simulink model "FullyConnectedMMG"  (R2020b)
settings: Solver=ode3  StartTime=0.0  StopTime=TimeS  FixedStep=Ts  RelTol=1e-3
values from neighbouring files (symbols this model uses):
  fr = 60    [MMG_Parameters.m]
  Lgs = 600e-6    (= 0.0006)    [MMG_Parameters.m]
  MaxWind = 18    [MMG_Parameters.m]
  MicroVol = 575    [MMG_Parameters.m]
  MinWind = 3    [MMG_Parameters.m]
  NomVol = 600    [MMG_Parameters.m]
  NomWind = 10    [MMG_Parameters.m]
  Pnombb = 400    [MMG_Parameters.m]
  PnomDG = 150e3    (= 150000)    [MMG_Parameters.m]
  PnomWT = 400e3    (= 400000)    [MMG_Parameters.m]
  Rgs = 20e-6    (= 2e-05)    [MMG_Parameters.m]
  RtCapM1 = (5.1)*1e-1    (= 0.51)    [MMG_Parameters.m]
  RtCapM2 = (5.1)*1e-1    (= 0.51)    [MMG_Parameters.m]
  SOC = [70,80,75,65]    [MMG_Parameters.m]
  Ts = 8e-4    (= 0.0008)    [MMG_Parameters.m]    (also in SolveMONO.m = 0.005)
  Vgrid = 25e3    (= 25000)    [MMG_Parameters.m]
  VMic = 575    [MMG_Parameters.m]
  Vs = 120e3    (= 120000)    [MMG_Parameters.m]
undefined symbols (not defined in the file or in its folder): DiscIntNeverNeededParam
libraries: powerlib x64, simulink x24, powerlib_meascontrol x16
(part 1 of 5)
settings Model: SimulationMode=accelerator  Creator=jlesage  LastModifiedBy=ferna
settings DataIOCC: ReturnWorkspaceOutputs=off
settings OptimizationCC: EfficientMapNaN2IntZero=off
settings DebuggingCC: UnconnectedInputMsg=none  UnconnectedOutputMsg=none  UnconnectedLineMsg=none  ArithmeticOperatorsInVariantConditions=warning
settings HardwareCC: TargetBitPerPointer=64  TargetBitPerSizeT=64  TargetBitPerPtrDiffT=64  TargetLongLongMode=on  TargetIntDivRoundTo=Zero  TargetEndianess=LittleEndian  TargetWordSize=64  TargetHWDeviceType=MATLAB Host  ProdEqTarget=off
settings SFSimCC: SimUseLocalCustomCode=off  CustomCodeUndefinedFunction=UseInterfaceOnly
settings CodeAppCC: MaxIdLength=128
settings GRTTargetCC: CombineOutputUpdateFcns=off  GRTInterface=on

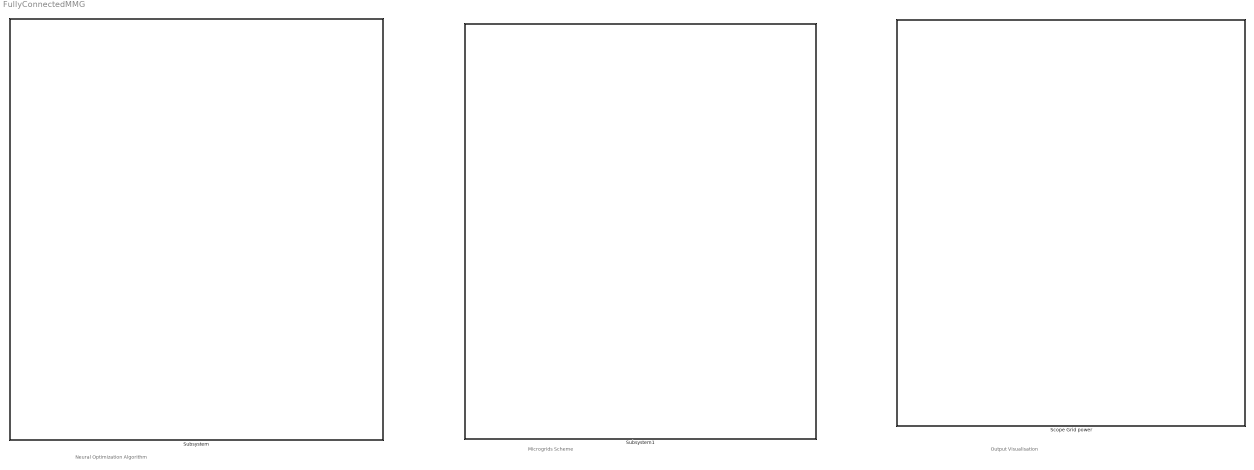
== system FullyConnectedMMG ==
  note: Output Visualisation
  note: Microgrids Scheme
  note: Neural Optimization Algorithm
  Scope Grid power : Subsystem
  Subsystem : Subsystem
  Subsystem1 : Subsystem

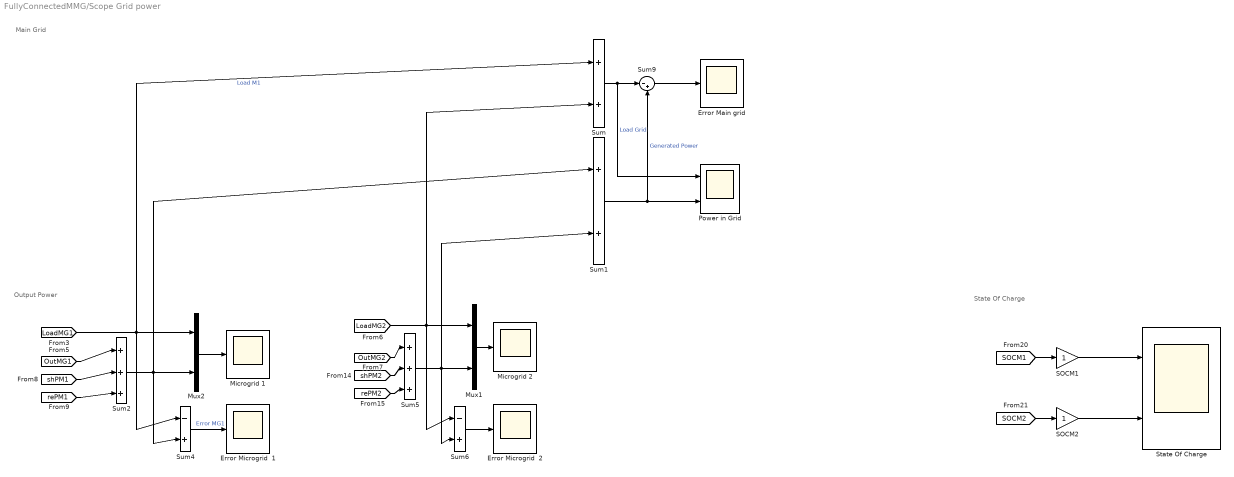
== system FullyConnectedMMG/Scope Grid power ==
  note: State Of Charge
  note: Output Power
  note: Main Grid
  Error Main grid : Scope
  Error Microgrid  1 : Scope
  Error Microgrid  2 : Scope
  Microgrid 1 : Scope
  Microgrid 2 : Scope
  Mux1 : Mux  Inputs=2
  Mux2 : Mux  Inputs=2
  Power in Grid : Scope  NumInputPorts=2
  SOCM1 : Gain
  SOCM2 : Gain
  State Of Charge : Scope  NumInputPorts=2
  Sum : Sum  Inputs=|++
  Sum1 : Sum  Inputs=|++
  Sum2 : Sum  Inputs=|+++
  Sum4 : Sum  Inputs=|-+
  Sum5 : Sum  Inputs=|+++
  Sum6 : Sum  Inputs=|-+
  Sum9 : Sum  Inputs=|-+
  wires:
  Sum5/1 -> Sum6/2, Mux1/2, Sum1/2
  Sum1/1 -> Power in Grid/2, Sum9/2  "Generated Power"
  Sum/1 -> Power in Grid/1, Sum9/1  "Load Grid"
  Mux2/1 -> Microgrid 1/1
  [LoadMG1] -> Sum/1, Mux2/1, Sum4/1  "Load M1"
  [LoadMG2] -> Sum6/1, Mux1/1, Sum/2
  Mux1/1 -> Microgrid 2/1
  Sum2/1 -> Sum4/2, Sum1/1, Mux2/2
  Sum4/1 -> Error Microgrid  1/1  "Error MG1"
  Sum6/1 -> Error Microgrid  2/1
  [SOCM1] -> SOCM1/1
  [SOCM2] -> SOCM2/1
  Sum9/1 -> Error Main grid/1
  SOCM1/1 -> State Of Charge/1
  SOCM2/1 -> State Of Charge/2
  [OutMG1] -> Sum2/1
  [OutMG2] -> Sum5/1
  [shPM1] -> Sum2/2
  [rePM1] -> Sum2/3
  [shPM2] -> Sum5/2
  [rePM2] -> Sum5/3

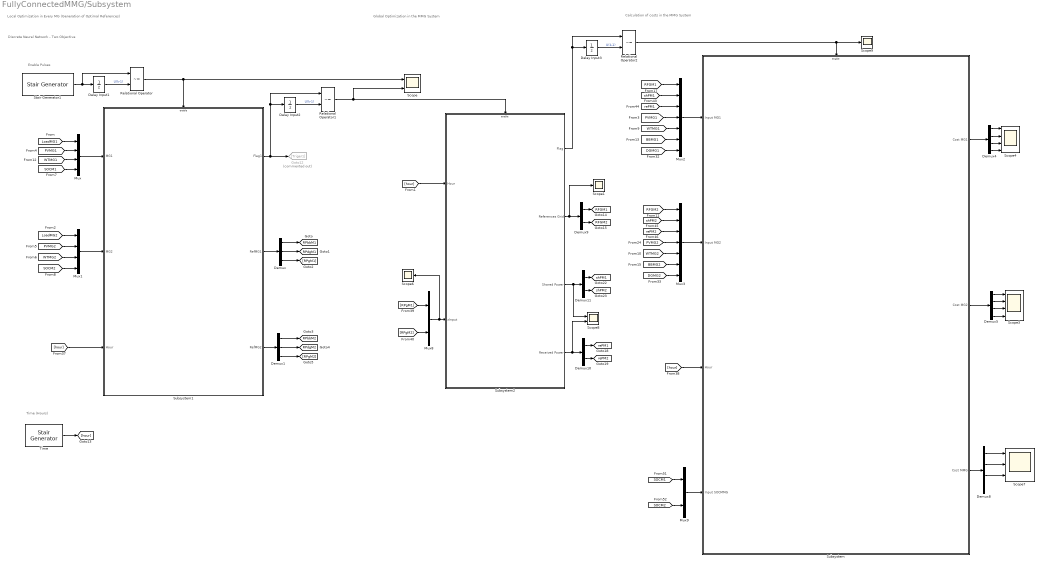
== system FullyConnectedMMG/Subsystem ==
  note: Enable Pulses
  note: Local Optimization in Every MG (Generation of Optimal References)
  note: Discrete Neural Network - Two Objective
  note: Calculation of costs in the MMG System
  note: Global Optimization in the MMG System
  note: Time (Hours)
  Delay Input1 : UnitDelay  Description=Store in Global RAM  DisableCoverage=on  SampleTime=-1  HasFrameUpgradeWarning=on
  Delay Input2 : UnitDelay  Description=Store in Global RAM  DisableCoverage=on  SampleTime=-1  HasFrameUpgradeWarning=on
  Delay Input3 : UnitDelay  Description=Store in Global RAM  DisableCoverage=on  SampleTime=-1  HasFrameUpgradeWarning=on
  Demux : Demux  Outputs=3
  Demux1 : Demux  Outputs=3
  Demux10 : Demux  Outputs=2
  Demux11 : Demux  Outputs=2
  Demux4 : Demux
  Demux5 : Demux
  Demux8 : Demux
  Demux9 : Demux  Outputs=2
  Goto12 : Goto  Commented=on  GotoTag=Triger1
  Mux : Mux
  Mux1 : Mux
  Mux2 : Mux  Inputs=7
  Mux3 : Mux  Inputs=7
  Mux8 : Mux  Inputs=2
  Mux9 : Mux  Inputs=2
  Relational Operator : RelationalOperator  Operator=~=  OutDataTypeStr=fixdt(0, 8)  ZeroCross=off  RndMeth=Nearest
  Relational Operator1 : RelationalOperator  Operator=~=  OutDataTypeStr=fixdt(0, 8)  ZeroCross=off  RndMeth=Nearest
  Relational Operator2 : RelationalOperator  Operator=~=  OutDataTypeStr=fixdt(0, 8)  ZeroCross=off  RndMeth=Nearest
  Scope : Scope  NumInputPorts=2
  Scope1 : Scope
  Scope3 : Scope  NumInputPorts=4
  Scope4 : Scope  NumInputPorts=4
  Scope6 : Scope
  Scope7 : Scope  NumInputPorts=3
  Scope8 : Scope  NumInputPorts=2
  Scope9 : Scope
  Stair Generator1 : powerlib_meascontrol/Pulse & Signal Generators/Stair Generator  t=[0, 1, 2, 3, 4, 5, 6, 7, 8, 9, 10, 11, 12, 13, 14, 15, 16, 17, 18, 19, 20, 21, 22, 23]+0.04  e=[1,2,3,4,5,6,7,8,9,10,11,12,13,14,15,16,17,18,19,20,21,22,23,24]  Ts=Ts
  Subsystem : Subsystem
  Subsystem1 : Subsystem
  Subsystem2 : Subsystem
  Time : powerlib_meascontrol/Pulse & Signal Generators/Stair Generator  t=[0.5,1.5,2.5,3.5,4.5,5.5,6.5,7.5,8.5,9.5,10.5,11.5,12.5,13.5,14.5,15.5,16.5,17.5,18.5,19.5,20.5,21.5,22.5,23.5]  e=[1,2,3,4,5,6,7,8,9,10,11,12,13,14,15,16,17,18,19,20,21,22,23,24]  Ts=0
  tag scope: RFGM1=global, RFGM2=global, RPbbM1=global, RPbbM2=global, RPdgM1=global, RPdgM2=global, rePM1=global, rePM2=global, shPM1=global, shPM2=global
  wires:
  Demux1/2 -> [RPdgM2]
  [SOCM2] -> Mux1/4
  Demux/1 -> [RPbbM1]
  [LoadMG1] -> Mux/1
  [PVMG1] -> Mux/2
  Demux/2 -> [RPdgM1]
  Demux1/3 -> [RPgM2]
  Demux1/1 -> [RPbbM2]
  [WTMG2] -> Mux1/3
  [PVMG2] -> Mux1/2
  [WTMG1] -> Mux/3
  [SOCM1] -> Mux/4
  Demux/3 -> [RPgM1]
  [LoadMG2] -> Mux1/1
  Mux2/1 -> Subsystem/1(Input MG1)
  [hour] -> Subsystem/3(Hour)
  Demux4/1 -> Scope4/1
  Demux4/2 -> Scope4/2
  Subsystem/1(Cost MG1) -> Demux4/1
  Demux5/2 -> Scope3/2
  Demux5/1 -> Scope3/1
  Subsystem/2(Cost MG2) -> Demux5/1
  Demux8/3 -> Scope7/3
  Demux8/1 -> Scope7/1
  Demux8/2 -> Scope7/2
  Subsystem/3(Cost MMG) -> Demux8/1
  Stair Generator1/1 -> Relational Operator/1, Delay Input1/1
  Delay Input1/1 -> Relational Operator/2  "U(k-1)"
  Relational Operator/1 -> Subsystem1/Enable, Scope/1
  Mux/1 -> Subsystem1/1(MG1)
  Mux1/1 -> Subsystem1/2(MG2)
  [hour] -> Subsystem1/3(Hour)
  Subsystem1/1(Flag1) -> Relational Operator1/1, Delay Input2/1, Goto12/1
  Subsystem1/2(RefMG1) -> Demux/1
  Subsystem1/3(RefMG2) -> Demux1/1
  Time/1 -> [hour]
  Relational Operator2/1 -> Scope9/1, Subsystem/Enable
  [RPgM1] -> Mux8/1
  [RPgM2] -> Mux8/2
  [hour] -> Subsystem2/1(Hour)
  Mux8/1 -> Scope6/1, Subsystem2/2(xInput)
  Delay Input2/1 -> Relational Operator1/2  "U(k-1)"
  Relational Operator1/1 -> Subsystem2/Enable, Scope/2
  Subsystem2/2(References Grid) -> Demux9/1, Scope1/1
  Demux9/1 -> [RFGM1]
  Demux9/2 -> [RFGM2]
  Demux10/2 -> [rePM2]
  Demux10/1 -> [rePM1]
  Subsystem2/3(Shared Power) -> Scope8/1, Demux11/1
  Subsystem2/4(Received Power) -> Scope8/2, Demux10/1
  Demux11/1 -> [shPM1]
  Demux11/2 -> [shPM2]
  [RFGM1] -> Mux2/1
  [rePM1] -> Mux2/3
  [shPM1] -> Mux2/2
  [PVMG1] -> Mux2/4
  [WTMG1] -> Mux2/5
  [BBMG1] -> Mux2/6
  [DGMG1] -> Mux2/7
  Mux3/1 -> Subsystem/2(Input MG2)
  [DGMG2] -> Mux3/7
  [BBMG2] -> Mux3/6
  [WTMG2] -> Mux3/5
  [PVMG2] -> Mux3/4
  [RFGM2] -> Mux3/1
  [shPM2] -> Mux3/2
  [rePM2] -> Mux3/3
  Delay Input3/1 -> Relational Operator2/2  "U(k-1)"
  Subsystem2/1(Flag) -> Delay Input3/1, Relational Operator2/1
  Mux9/1 -> Subsystem/4(Input SOCMMG)
  [SOCM2] -> Mux9/2
  [SOCM1] -> Mux9/1
  Demux4/3 -> Scope4/3
  Demux5/3 -> Scope3/3
  Demux4/4 -> Scope4/4
  Demux5/4 -> Scope3/4

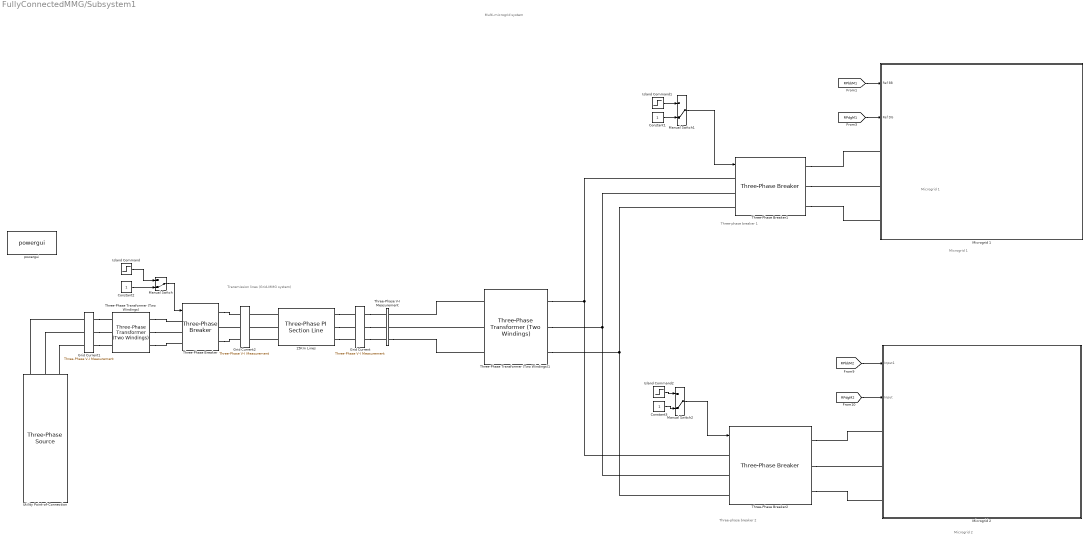
== system FullyConnectedMMG/Subsystem1 ==
  note: Three-phase breaker 1
  note: Microgrid 2
  note: Three-phase breaker 2
  note: Microgrid 1
  note: Transmission lines (Grid-MMG system)
  note: Microgrid 1
  note: Multi-microgrid system
  15Km Lines : powerlib/Elements/Three-Phase PI Section Line  LConnTagsString=a|b|c  RConnTagsString=A|B|C  Length=15  Frequency=fr  Resistances=[0.25 0.413]  Inductances=[1.05e-3 3.32e-3]  Capacitances=[11.33e-009 5.01e-009]
  Constant1 : Constant
  Constant2 : Constant
  Constant3 : Constant
  Grid Current : powerlib/Measurements/Three-Phase V-I Measurement  VoltageMeasurement=phase-to-ground  SetLabelV=on  LabelV=Vabc_g  Vpu=off  VpuLL=off  CurrentMeasurement=yes  SetLabelI=on  LabelI=Iabc_sg  Ipu=off  Pbase=100e6  Vbase=500e3  OutputType=Complex  PhasorSimulation=off  PSBequivalent=0
  Grid Current1 : powerlib/Measurements/Three-Phase V-I Measurement  VoltageMeasurement=phase-to-ground  SetLabelV=on  LabelV=Vabc1  Vpu=off  VpuLL=off  CurrentMeasurement=yes  SetLabelI=on  LabelI=Iabc1  Ipu=off  Pbase=100e6  Vbase=500e3  OutputType=Complex  PhasorSimulation=off  PSBequivalent=0
  Grid Current2 : powerlib/Measurements/Three-Phase V-I Measurement  VoltageMeasurement=phase-to-ground  SetLabelV=on  LabelV=VabcGrid  Vpu=off  VpuLL=off  CurrentMeasurement=yes  SetLabelI=on  LabelI=IabcGrid  Ipu=off  Pbase=100e6  Vbase=500e3  OutputType=Complex  PhasorSimulation=off  PSBequivalent=0
  Island Command : Step  Time=15  Before=1  After=0  SampleTime=0
  Island Command1 : Step  Time=7  SampleTime=0
  Island Command2 : Step  Time=7  SampleTime=0
  Manual Switch : ManualSwitch  CurrentSetting=0
  Manual Switch1 : ManualSwitch  CurrentSetting=0
  Manual Switch2 : ManualSwitch  CurrentSetting=0
  Microgrid 1 : Subsystem
      mask Display:
      | % image('C:\Users\ferna\OneDrive\Escritorio\Neural-Simulations\Working-IN\Multi-Micro\MMG_Working_4MGs\Images\generic-microgrid.jpg'); % Use "Edit Image" on toolstrip to change.
      | % image('C:\Users\CINVESTAV\OneDrive\Escritorio\Neural-Simulations\Working-IN\Multi-Micro\MMG_Working_4MGs\Images\generic-microgrid.jpg');
      | 
      | image(imread('MG.jpg'));
  Microgrid 2 : Subsystem
      mask Display:
      | % image('C:\Users\CINVESTAV\OneDrive\Escritorio\Neural-Simulations\Working-IN\Multi-Micro\MMG_Working_4MGs\Images\generic-microgrid.jpg'); % Use "Edit Image" on toolstrip to change.
      | % image('C:\Users\ferna\OneDrive\Escritorio\Neural-Simulations\Working-IN\Multi-Micro\MMG_Working_4MGs\Images\generic-microgrid.jpg'); % Use "Edit Image" on toolstrip to change.
      | 
      | image(imread('MG.jpg'));
  Three-Phase Transformer (Two Windings) : powerlib/Elements/Three-Phase Transformer (Two Windings)  Winding1Connection=Yg  Winding2Connection=Yg  CoreType=Three single-phase transformers  SetSaturation=off  Hysteresis=off  DataFile='hysteresis'  SetInitialFlux=off  Measurements=None  UNITS=pu  NominalPower=[ 250e6 , fr]  Winding1=[Vs , 0.002 , 0.08 ]  Winding2=[Vgrid , 0.002 , 0.08 ]  Rm=500  Lm=500  L0=0.5  Saturation=[ 0,0 ; 0.0024,1.2 ; 1.0,1.52 ]  InitialFluxes=[ 0.8 , -0.8 , 0.7 ]  BreakLoop=off  DiscreteSolver=Trapezoidal iterative  DataType=off  TransfoNumber=1
  Three-Phase Transformer (Two Windings)1 : powerlib/Elements/Three-Phase Transformer (Two Windings)  Winding1Connection=Yg  Winding2Connection=Yg  CoreType=Three single-phase transformers  SetSaturation=off  Hysteresis=off  DataFile='hysteresis'  SetInitialFlux=off  Measurements=None  UNITS=pu  NominalPower=[ 25e6 , 60 ]  Winding1=[25e3 , 0.002 , 0.08 ]  Winding2=[575 , 0.002 , 0.08 ]  Rm=500  Lm=500  L0=0.5  Saturation=[ 0,0 ; 0.0024,1.2 ; 1.0,1.52 ]  InitialFluxes=[ 0.8 , -0.8 , 0.7 ]  BreakLoop=off  DiscreteSolver=Trapezoidal iterative  DataType=off  TransfoNumber=1
  Three-Phase V-I Measurement : powerlib/Measurements/Three-Phase V-I Measurement  VoltageMeasurement=phase-to-ground  SetLabelV=on  LabelV=Vabc  Vpu=off  VpuLL=off  CurrentMeasurement=yes  SetLabelI=on  LabelI=Iabc  Ipu=off  Pbase=100e6  Vbase=500e3  OutputType=Complex  PhasorSimulation=off  PSBequivalent=0
  Three-Phase Breaker : powerlib/Elements/Three-Phase Breaker  InitialState=closed  SwitchA=on  SwitchB=on  SwitchC=on  SwitchTimes="[1/60  5/60]"  External=on  BreakerResistance=0.01  SnubberResistance=1e6  SnubberCapacitance=inf  Measurements=None
  Three-Phase Breaker1 : powerlib/Elements/Three-Phase Breaker  InitialState=closed  SwitchA=on  SwitchB=on  SwitchC=on  SwitchTimes="[1/60  5/60]"  External=on  BreakerResistance=0.01  SnubberResistance=1e6  SnubberCapacitance=inf  Measurements=None
  Three-Phase Breaker2 : powerlib/Elements/Three-Phase Breaker  InitialState=closed  SwitchA=on  SwitchB=on  SwitchC=on  SwitchTimes="[1/60  5/60]"  External=on  BreakerResistance=0.01  SnubberResistance=1e6  SnubberCapacitance=inf  Measurements=None
  Utility Point-of-Connection : powerlib/Electrical Sources/Three-Phase Source  InternalConnection=Yg  VoltagePhases=off  Voltage=Vs  PhaseAngle=0.071468  Voltage_phases=[25e3 25e3 25e3]/sqrt(3)  PhaseAngles_phases=[0 -120 +120]  Frequency=60  NonIdealSource=on  SpecifyImpedance=on  Resistance=0.8929  Inductance=16.58e-3  ShortCircuitLevel=250e6  BaseVoltage=13.8e3  XRratio=7  BusType=swing  Pref=10e3  Qref=0  Prefabc=[10e3, 10e3, 10e3]  Qrefabc=[0, 0, 0]  Qmin=-inf  Qmax=inf
  powergui : powerlib/powergui  Priority=1  SimulationMode=Discrete  SampleTime=Ts  frequency=60  Iterations=50  frequencyindice=60  Pbase=100e6  ErrMax=0.0001  UnitsV=kV  UnitsW=MW  buscounter=3  FunctionMessages=off  echomessages=off  EnableUseOfTLC=off  CurrentSourceSwitches=off  DisableSnubberDevices=off  DisableRonSwitches=off  DisableVfSwitches=off  DisplayEquations=off  AutomaticDiscreteSolvers=off  SolverType=Tustin/Backward Euler (TBE)  Interpol=off  ExternalGateDelay=off  methode=off  Ts=100  x0status=blocks  SPID=on  SwTol=0  HookPort=off  NonlinearTolerance=1e-4  nMaxIteration=100  ContinueOnMaxIteration=off  RestoreLinks=warning  ResistiveCurrentMeasurement=off  Frange=[0:2:500]  Ylog=off  Xlog=on  ShowGrid=off  save=off  variable=ZData  structure=0  ZoomFFT=off  StartTime=0.0  cycles=1  DisplayStyle=1  fundamental=60  FreqAxis=off  MaxFrequency=1000  frequencyindicesteady=1  RmsSteady=1  display=off
  wires:
  [RPdgM1] -> Microgrid 1/2(Ref DG)
  Manual Switch1/1 -> Three-Phase Breaker1/1
  [RPdgM2] -> Microgrid 2/2(Input)
  Constant1/1 -> Manual Switch1/2
  Manual Switch2/1 -> Three-Phase Breaker2/1
  [RPbbM2] -> Microgrid 2/1(Input1)
  Constant3/1 -> Manual Switch2/2
  Manual Switch/1 -> Three-Phase Breaker/1
  [RPbbM1] -> Microgrid 1/1(Ref BB)
  Island Command2/1 -> Manual Switch2/1
  Island Command/1 -> Manual Switch/1
  Constant2/1 -> Manual Switch/2
  Island Command1/1 -> Manual Switch1/1
  connections:
  Grid Current1/LConn3 -- Three-Phase Transformer (Two Windings)/LConn3
  Grid Current/LConn1 -- Three-Phase V-I Measurement/LConn1
  Grid Current2/LConn2 -- Three-Phase Breaker/RConn2
  15Km Lines/LConn2 -- Grid Current2/RConn2
  Three-Phase Breaker1/RConn1 -- Microgrid 1/LConn1
  Three-Phase Breaker2/RConn1 -- Microgrid 2/LConn1
  Grid Current1/LConn2 -- Three-Phase Transformer (Two Windings)/LConn2
  Three-Phase Transformer (Two Windings)/RConn2 -- Three-Phase Breaker/LConn2
  Grid Current1/RConn3 -- Utility Point-of-Connection/RConn3
  15Km Lines/LConn3 -- Grid Current2/RConn3
  Grid Current/LConn3 -- Three-Phase V-I Measurement/LConn3
  Three-Phase Breaker/RConn3 -- Grid Current2/LConn3
  Three-Phase Breaker2/LConn1 -- Three-Phase Breaker1/LConn1 -- Three-Phase Transformer (Two Windings)1/RConn1
  Three-Phase Breaker2/LConn2 -- Three-Phase Breaker1/LConn2 -- Three-Phase Transformer (Two Windings)1/RConn2
  Grid Current1/LConn1 -- Three-Phase Transformer (Two Windings)/LConn1
  Three-Phase Transformer (Two Windings)/RConn3 -- Three-Phase Breaker/LConn3
  15Km Lines/RConn3 -- Grid Current/RConn3
  Three-Phase Transformer (Two Windings)/RConn1 -- Three-Phase Breaker/LConn1
  Three-Phase Breaker2/RConn2 -- Microgrid 2/LConn2
  Three-Phase Breaker2/RConn3 -- Microgrid 2/LConn3
  15Km Lines/RConn2 -- Grid Current/RConn2
  Grid Current1/RConn2 -- Utility Point-of-Connection/RConn2
  Grid Current1/RConn1 -- Utility Point-of-Connection/RConn1
  Three-Phase Breaker2/LConn3 -- Three-Phase Breaker1/LConn3 -- Three-Phase Transformer (Two Windings)1/RConn3
  Grid Current/LConn2 -- Three-Phase V-I Measurement/LConn2
  Three-Phase Breaker1/RConn2 -- Microgrid 1/LConn2
  15Km Lines/RConn1 -- Grid Current/RConn1
  Three-Phase Breaker/RConn1 -- Grid Current2/LConn1
  Three-Phase Breaker1/RConn3 -- Microgrid 1/LConn3
  15Km Lines/LConn1 -- Grid Current2/RConn1
  Three-Phase Transformer (Two Windings)1/LConn2 -- Three-Phase V-I Measurement/RConn2
  Three-Phase Transformer (Two Windings)1/LConn1 -- Three-Phase V-I Measurement/RConn1
  Three-Phase V-I Measurement/RConn3 -- Three-Phase Transformer (Two Windings)1/LConn3

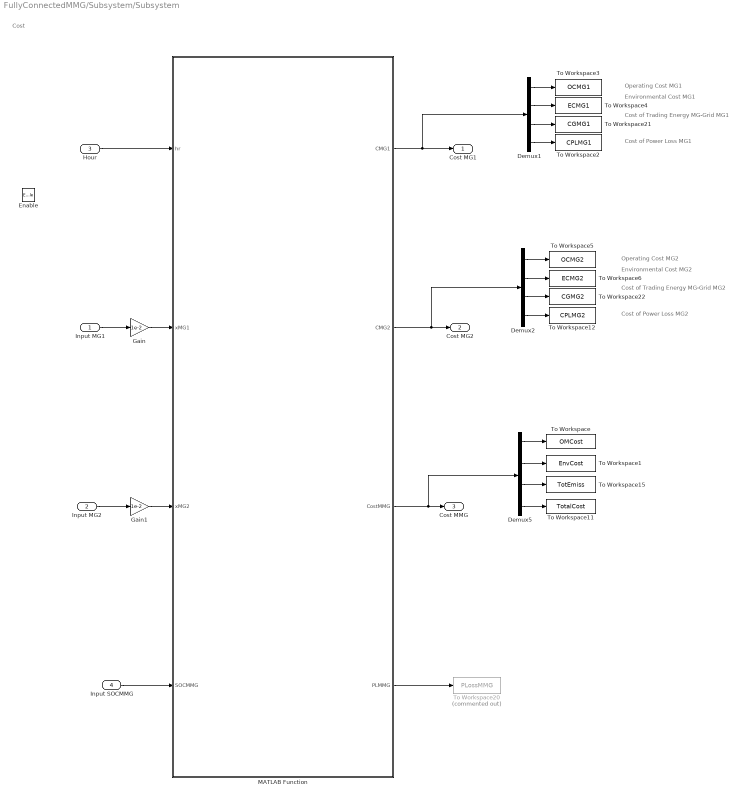
== system FullyConnectedMMG/Subsystem/Subsystem ==
  note: Operating Cost MG1
  note: Cost
  note: Environmental Cost MG1
  note: Cost of Trading Energy MG-Grid MG1
  note: Cost of Power Loss MG1
  note: Operating Cost MG2
  note: Cost of Trading Energy MG-Grid MG2
  note: Environmental Cost MG2
  note: Cost of Power Loss MG2
  Input MG1 : Inport
  Input MG2 : Inport  Port=2
  Hour : Inport  Port=3
  Input SOCMMG : Inport  Port=4
  Enable : EnablePort
  Demux1 : Demux
  Demux2 : Demux
  Demux5 : Demux
  Gain : Gain  Gain=1e-2
  Gain1 : Gain  Gain=1e-2
  MATLAB Function : MATLAB Function  TreatAsAtomicUnit=on
  To Workspace : ToWorkspace  VariableName=OMCost  SampleTime=Ts
      settings: Save2DSignal=2-D array (concatenate along first dimension)
  To Workspace1 : ToWorkspace  VariableName=EnvCost  SampleTime=Ts
      settings: Save2DSignal=2-D array (concatenate along first dimension)
  To Workspace11 : ToWorkspace  VariableName=TotalCost  SampleTime=Ts
      settings: Save2DSignal=2-D array (concatenate along first dimension)
  To Workspace12 : ToWorkspace  VariableName=CPLMG2  SampleTime=Ts
      settings: Save2DSignal=2-D array (concatenate along first dimension)
  To Workspace15 : ToWorkspace  VariableName=TotEmiss  SampleTime=Ts
      settings: Save2DSignal=2-D array (concatenate along first dimension)
  To Workspace2 : ToWorkspace  VariableName=CPLMG1  SampleTime=Ts
      settings: Save2DSignal=2-D array (concatenate along first dimension)
  To Workspace20 : ToWorkspace  Commented=on  VariableName=PLossMMG  SampleTime=Ts
      settings: Save2DSignal=2-D array (concatenate along first dimension)
  To Workspace21 : ToWorkspace  VariableName=CGMG1  SampleTime=Ts
      settings: Save2DSignal=2-D array (concatenate along first dimension)
  To Workspace22 : ToWorkspace  VariableName=CGMG2  SampleTime=Ts
      settings: Save2DSignal=2-D array (concatenate along first dimension)
  To Workspace3 : ToWorkspace  VariableName=OCMG1  SampleTime=Ts
      settings: Save2DSignal=2-D array (concatenate along first dimension)
  To Workspace4 : ToWorkspace  VariableName=ECMG1  SampleTime=Ts
      settings: Save2DSignal=2-D array (concatenate along first dimension)
  To Workspace5 : ToWorkspace  VariableName=OCMG2  SampleTime=Ts
      settings: Save2DSignal=2-D array (concatenate along first dimension)
  To Workspace6 : ToWorkspace  VariableName=ECMG2  SampleTime=Ts
      settings: Save2DSignal=2-D array (concatenate along first dimension)
  Cost MG1 : Outport
  Cost MG2 : Outport  Port=2
  Cost MMG : Outport  Port=3
  wires:
  Input MG1/1 -> Gain/1
  Input MG2/1 -> Gain1/1
  Hour/1 -> MATLAB Function/1(hr)
  MATLAB Function/2(CMG2) -> Demux2/1, Cost MG2/1
  Demux2/1 -> To Workspace5/1
  MATLAB Function/1(CMG1) -> Demux1/1, Cost MG1/1
  Demux1/1 -> To Workspace3/1
  Demux5/1 -> To Workspace/1
  Demux5/2 -> To Workspace1/1
  MATLAB Function/3(CostMMG) -> Demux5/1, Cost MMG/1
  Gain/1 -> MATLAB Function/2(xMG1)
  Gain1/1 -> MATLAB Function/3(xMG2)
  Demux2/4 -> To Workspace12/1
  Demux1/4 -> To Workspace2/1
  MATLAB Function/4(PLMMG) -> To Workspace20/1
  Input SOCMMG/1 -> MATLAB Function/4(SOCMMG)
  Demux1/2 -> To Workspace4/1
  Demux1/3 -> To Workspace21/1
  Demux2/2 -> To Workspace6/1
  Demux2/3 -> To Workspace22/1
  Demux5/4 -> To Workspace11/1
  Demux5/3 -> To Workspace15/1

== system FullyConnectedMMG/Subsystem/Subsystem1 ==
  MG1 : Inport
  MG2 : Inport  Port=2
  Hour : Inport  Port=3
  Enable : EnablePort
  Neural Network Optimization : MATLAB Function  TreatAsAtomicUnit=on
  Flag1 : Outport
  RefMG1 : Outport  Port=2
  RefMG2 : Outport  Port=3
  wires:
  Hour/1 -> Neural Network Optimization/3(hour)
  Neural Network Optimization/3(RefMG2) -> RefMG2/1
  Neural Network Optimization/1(Flag1) -> Flag1/1
  MG2/1 -> Neural Network Optimization/2(MG2)
  Neural Network Optimization/2(RefMG1) -> RefMG1/1
  MG1/1 -> Neural Network Optimization/1(MG1)

== system FullyConnectedMMG/Subsystem/Subsystem2 ==
  Hour : Inport
  xInput : Inport  Port=2
  Enable : EnablePort
  MATLAB Function : MATLAB Function  TreatAsAtomicUnit=on
  Flag : Outport
  References Grid : Outport  Port=2
  Shared Power : Outport  Port=3
  Received Power : Outport  Port=4
  wires:
  Hour/1 -> MATLAB Function/1(Hour)
  xInput/1 -> MATLAB Function/2(xInput)
  MATLAB Function/4(Flag) -> Flag/1
  MATLAB Function/1(outGrid) -> References Grid/1
  MATLAB Function/2(shMGs) -> Shared Power/1
  MATLAB Function/3(recMGs) -> Received Power/1

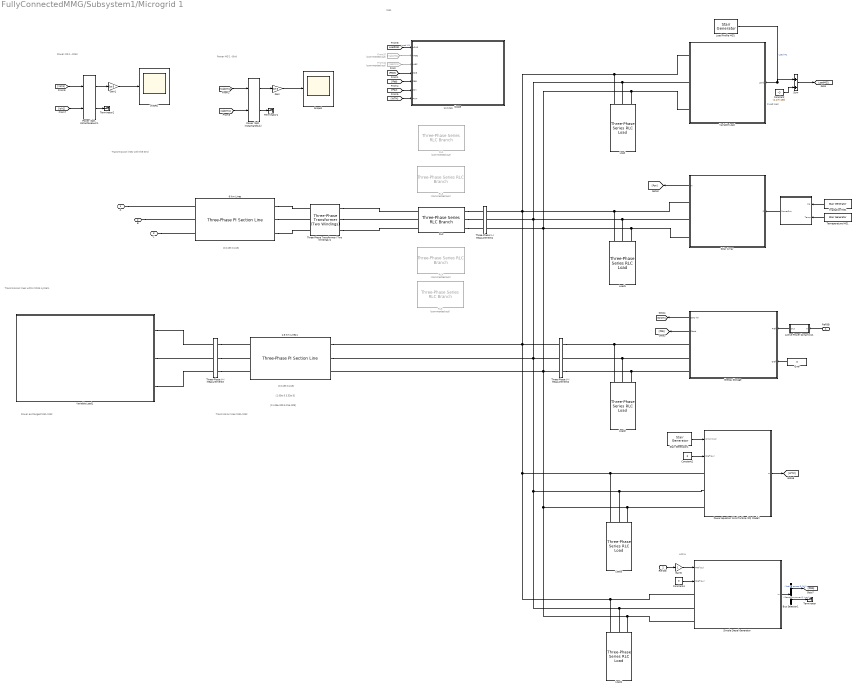
== system FullyConnectedMMG/Subsystem1/Microgrid 1 ==
  note: [11.33e-009 5.01e-009]
  note: [1.05e-3 3.32e-3]
  note: [0.1153 0.413]
  note: Fixed load
  note: SCOPES
  note: w2Kw
  note: MG1
  note: Power MG 1 -MGm
  note: Transmission lines with the Grid
  note: Transmission lines within MMG system
  note: [0.1153 0.413]
  note: Tranmission lines MG1-MG2
  note: Power exchanged MG1-MG2
  note: Power MG 1 -Grid
  Ref BB : Inport
  Ref DG : Inport  Port=2
  " " : Subsystem  VariantControl=T6NotZero  mask{Pvr=200, Dfac=0.98, Tfac=0.3, Tsc=25}
      mask prompts: Pvr "Rated Power (kW)"; Dfac "Derating Factor"; Tfac "Temperature Factor"; Tsc "Standard Temperature (C)"
  1.5 Km Lines1 : powerlib/Elements/Three-Phase PI Section Line  LConnTagsString=a|b|c  RConnTagsString=A|B|C  Length=1.5  Frequency=fr  Resistances=[0.1153 0.413]  Inductances=[1.05e-3 3.32e-3]  Capacitances=[11.33e-009 5.01e-009]
  6 Km Lines : powerlib/Elements/Three-Phase PI Section Line  LConnTagsString=a|b|c  RConnTagsString=A|B|C  Length=6  Frequency=fr  Resistances=[0.0153 0.413]  Inductances=[1.05e-3 3.32e-3]  Capacitances=[11.33e-009 5.01e-009]
  Active Power Dynamics1 : Subsystem  VariantControl=T6NotZero
      mask Display: disp('1 / (1 + s T_P)','texmode','on');
  Bus Selector1 : BusSelector  OutputSignals=Active power P (W),Reactive power Q (var)
  Constant : Constant  Value=(2.1)*(1e3)
  Constant2 : Constant  Value=0
  Constant4 : Constant  Value=0
  Energy Storage : Subsystem  mask(Grid-connected Energy Storage (PQ Model)){Vn=NomVol, Fn=60, PnomkW=Pnombb, kWh_Rated=RtCapM1, Efficiency=96, LimitVec=[90 10], RechargeSOC=11, Precharge=50, autoRecharge=off, Initial_kWh_pc=SOC(1), PQvec=[500e3 0], Ts=Ts}
      mask prompts: Vn "Nominal L-L Voltage [Vrms]"; Fn "Nominal Frequency [Hz]"; PnomkW "Rated Power [kW]"; kWh_Rated "Rated Capacity [kWh]"; Efficiency "Overall System Efficiency [%]"; LimitVec "Upper/Lower Charge Limits [%]"; RechargeSOC "SOC to Recharge [%]"; Precharge "Recharge Rate [% of Rated Power]"; autoRecharge "Enable Auto-Recharge"; Initial_kWh_pc "Initial State-of-Charge [0-100%]"; PQvec "Initial Active/Reactive Cmds"; Ts "Sample Time"
      mask help:
      | The energy storage block models a generic grid-connected energy storage system (ESS), most commonly a battery system. This is a system-level model that does not contain any power electronics, but is useful for load flow, phasor, and hybrid phasor-EMT simulations. The inputs to this block are the commanded active and reactive power of the ESS. The ESS is assumed to have four quadrent operation.
      |
      | For more detailed ESS models, consider the battery block in the Drives library. Consider using this PQ Model to perform load flow studies and switch to a more detailed model when full EMT studies or more advanced controls are required.
      |
      | Note: The initial active/reactive power commands must be specified for use for Load Flow analysis.
      mask init:
      | % Calculate Initial Conditions
      | Pnom = PnomkW*1e3;
      | P0 = -PQvec(1);  Q0 = -PQvec(2);
      | if abs(P0) > Pnom
      |     P0 = sign(P0)*Pnom;
      | end
      | 
      | % Calculate Q0 given Reactive Power Capability Curve
      | Qlim = sqrt(Pnom^2 - P0^2);
      | if Qlim > abs(Q0)
      |     Q0 = sign(Q0)*Qlim;
      | end
      | 
      | UpChrgLim = LimitVec(1);
      | LowChrgLim = LimitVec(2);
      | if Initial_kWh_pc > UpChrgLim && P0 < 0
      |     P0 = 0; Q0 = 0;
      | elseif Initial_kWh_pc < LowChrgLim && P0 > 0
      |     P0 = 0; Q0 = 0;
      | end
      mask DialogControl Container7 Prompt: Grid Connection Properties
      mask DialogControl Container11 Prompt: Charge/Discharge Controls
      mask DialogControl Container12 Prompt: Initial Conditions
      mask Display: image(imread('Battery.png'))
  From34 : From  Commented=on  GotoTag=IabcM1  TagVisibility=global
      settings: CloseFcn=tagdialog Close
  From37 : From  Commented=on  GotoTag=VabcM1  TagVisibility=global
      settings: CloseFcn=tagdialog Close
  Gain : Gain  Gain=1e-3
  Gain1 : Gain  Gain=1e-3
  Gain5 : Gain
  Irradiation MG1 : powerlib_meascontrol/Pulse & Signal Generators/Stair Generator  t=Time  e=IrMG1  Ts=Ts
  Load{,1..4} (5 alike) : powerlib/Elements/Three-Phase Series RLC Load  LConnTagsString=A|B|C  Configuration=Y (grounded)  NominalVoltage=575  Vabc=[1e3 1e3 1e3]  Vabcp=[1e3 1e3 1e3]  NominalFrequency=60  UnbalancedPower=off  ActivePower=1e3  InductivePower=0  CapacitivePower=0  Pabc=[10e3 9e3 11e3]  QLabc=[100 90 110]  QCabc=[100 90 110]  Pabcp=[10e3 9e3 11e3]  QLabcp=[100 90 110]  QCabcp=[100 90 110]  Measurements=None  LoadType=constant Z
      settings: AttributesFormatString=P = %<ActivePower> W
  Load Profile MG1 : powerlib_meascontrol/Pulse & Signal Generators/Stair Generator  t=Time  e=PLoad1  Ts=Ts
  "Power (3ph, Instantaneous)" : powerlib_meascontrol/Measurements/Power (3ph, Instantaneous)
  "Power (3ph, Instantaneous)1" : powerlib_meascontrol/Measurements/Power (3ph, Instantaneous)
  Power Equation Wind Turbine (PQ Model) : Subsystem  AncestorBlock=|  mask{Unom=NomWind, Umax=MaxWind, Umin=MinWind, Pselect=Simple Cubic Power, rp=7, Cp=16/27, rho=1.225, Pnom=PnomWT, Uvec=[1:1:30], Pvec=[0,0,0,0,21359.3750000000,58193.5000000000,104316.125000000,157104.500000000,213935.875000000,272187.500000000,329236.625000000,382460.500000000,429236.375000000,466941.500000000,492953.125000000,500000,500000,500000,500000,500000,500000,500000,500000,500000,500000,0,0,0,0,0]*1e-1, Tp=0.1, Tq=1, ReactP=30}
      | exampleMicrogridLibrary/Power Equation
      | Wind Turbine
      | (PQ Model)
      mask prompts: Unom "Nominal Wind Speed [m/s]"; Umax "Maximum Operating Wind [m/s]"; Umin "Minimum Operating Wind [m/s]"; Pselect "Wind Turbine Power Method"; rp "Blade Radius, r [m]"; Cp "Performance Coefficient, Cp"; rho "Air Density, rho [kg/m^3]"; Pnom "Nominal Power, [W]"; Uvec "Wind Vec [m/s]"; Pvec "Power Vec [W]"; Tp "Active Power Dynamics, Tp [s]"; Tq "Reactive Power Dynamics, Tq [s]"; ReactP "Reactive Power Percentage [%]"
      mask help:
      | Simple Wind Turbine that serves as an Active and Reactive Power Source depending on the Wind Power Curve.
      |
      | The Wind Turbine Power Curve can be defined by:
      | - Dimentions of the wind turbine
      | - Simple cubic power curve
      | - Look-up vector from a wind turbine data sheet.
      mask init:
      | A = pi*rp^2;
      | 
      | if Pselect == 1,
      |     Pmax = 1/2*rho*Cp*A*Umax^3;
      | elseif Pselect == 2,
      |     Pmax = Pnom;
      | else
      |     Pmax = max(Pvec);
      | end
      | Qmax = ReactP/100*Pmax;
      mask TypeOptions Pselect: Using Properties | Simple Cubic Power | Look-up Fit
      mask DialogControl Container4 Prompt: General
      mask DialogControl Container9 Prompt: Dimensions
      mask DialogControl Container12 Prompt: Cubic
      mask DialogControl Container7 Prompt: Lookup
      mask DialogControl Container8 Prompt: Dynamics
      mask Display:
      | image(imread('eolienne.bmp'))
      | 
      | color('white')
      | port_label('LConn',1,'A')
      | port_label('LConn',2,'B')
      | port_label('LConn',3,'C')
      | 
      | color('blue')
      | port_label('output',1,'m')
      | port_label('input',1,'Wind (m/s)')
      | port_label('input',2,'Qref')
  Qref : Constant  Value=0
  RL{1,3..5} (4 alike) : powerlib/Elements/Three-Phase Series RLC Branch  Commented=on  LConnTagsString=A|B|C  RConnTagsString=A|B|C  BranchType=RL  Resistance=Rgs  Inductance=Lgs  Capacitance=inf  Measurements=None
  RL2 : powerlib/Elements/Three-Phase Series RLC Branch  LConnTagsString=A|B|C  RConnTagsString=A|B|C  BranchType=RL  Resistance=Rgs  Inductance=500e-6  Capacitance=inf  Measurements=None
  Scope : Subsystem
  Scope1 : Scope
  Scope2 : Scope
  Simple Diesel Generator : Subsystem  AncestorBlock=|  mask{Pn=PnomDG, Vn=VMic, Fn=fr, Tp=0.1, Tq=1, ReactP=30}
      | exampleMicrogridLibrary/Power Equation
      | Wind Turbine
      | (PQ Model)
      mask prompts: Pn "Generator Rated Power [W]"; Vn "Rated Voltage [V]"; Fn "Rated Frequency [Hz]"; Tp "Active Power Dynamics, Tp [s]"; Tq "Reactive Power Dynamics, Tq [s]"; ReactP "Reactive Power Percentage [%]"
      mask help:
      | Simple Wind Turbine that serves as an Active and Reactive Power Source depending on the Wind Power Curve.
      |
      | The Wind Turbine Power Curve can be defined by:
      | - Dimentions of the wind turbine
      | - Simple cubic power curve
      | - Look-up vector from a wind turbine data sheet.
      mask init:
      | Pmax = 320e3;
      | Qmax = ReactP/100*Pmax;
      mask DialogControl Container4 Prompt: General
      mask DialogControl Container8 Prompt: Dynamics
      mask Display:
      | image(imread('DGEN.jpg'));
      | color('black')
  Solar Array : Subsystem  mask(Grid-Connected PV Array (PQ Model)){Vn=MicroVol, Fn=fr, P0=500e3}
      mask prompts: Vn "Nominal L-L Voltage [Vrms]"; Fn "Nominal Frequency [Hz]"; P0 "Initial Power [W]"
      mask help:
      | This block models a grid-connected solar array using the Three-Phase Dynamic Load block. This is a system-level model that does not contain any power electronics, but is useful for load flow, phasor, and hybrid phasor-EMT simulations. The input to this block is the power output of the grid connected PV array, not irradiance.
      |
      | For more detailed PV models, consider the PV Array block in the Renewables library. Consider using this PQ Model to perform load flow studies and switch to a more detailed model when full EMT studies are required.
      |
      | Note: The array power must be specified for use for Load Flow analysis.
      mask init:
      | % P0 = Irr0*TotalArea*Efficiency/100;
      | P0 = -P0;
      mask Display:
      | image(imread('PV_Farm.jpg'))
      | color('white')
      | port_label('input',1,'P')
      | port_label('output',1,'m')
      | port_label('Rconn',1,'A')
      | port_label('Rconn',2,'B')
      | port_label('Rconn',3,'C')
  Stair Generator1 : powerlib_meascontrol/Pulse & Signal Generators/Stair Generator  t=Time  e=WindM1  Ts=Ts
  Sum : Sum  Inputs=|++
  Temeperature MG1 : powerlib_meascontrol/Pulse & Signal Generators/Stair Generator  t=Time  e=TempMG1  Ts=Ts
  Terminator : Terminator
  Terminator1 : Terminator
  Terminator2 : Terminator
  Three-Phase Transformer (Two Windings)1 : powerlib/Elements/Three-Phase Transformer (Two Windings)  Winding1Connection=Yg  Winding2Connection=Yg  CoreType=Three single-phase transformers  SetSaturation=off  Hysteresis=off  DataFile='hysteresis'  SetInitialFlux=off  Measurements=None  UNITS=pu  NominalPower=[ 25e6 , 60 ]  Winding1=[575 , 0.002 , 0.08 ]  Winding2=[575 , 0.002 , 0.08 ]  Rm=500  Lm=1500  L0=0.5  Saturation=[ 0,0 ; 0.0024,1.2 ; 1.0,1.52 ]  InitialFluxes=[ 0.8 , -0.8 , 0.7 ]  BreakLoop=off  DiscreteSolver=Trapezoidal iterative  DataType=off  TransfoNumber=1
  Three-Phase V-I Measurement1 : powerlib/Measurements/Three-Phase V-I Measurement  VoltageMeasurement=phase-to-ground  SetLabelV=on  LabelV=VabcM1  Vpu=off  VpuLL=off  CurrentMeasurement=yes  SetLabelI=on  LabelI=IabcM1  Ipu=off  Pbase=100e6  Vbase=500e3  OutputType=Complex  PhasorSimulation=off  PSBequivalent=0
  Three-Phase V-I Measurement2 : powerlib/Measurements/Three-Phase V-I Measurement  VoltageMeasurement=phase-to-ground  SetLabelV=on  LabelV=Vbb1  Vpu=off  VpuLL=off  CurrentMeasurement=yes  SetLabelI=on  LabelI=Ibb1  Ipu=off  Pbase=100e6  Vbase=500e3  OutputType=Complex  PhasorSimulation=off  PSBequivalent=0
  Three-Phase V-I Measurement3 : powerlib/Measurements/Three-Phase V-I Measurement  VoltageMeasurement=phase-to-ground  SetLabelV=on  LabelV=Vsh1  Vpu=off  VpuLL=off  CurrentMeasurement=yes  SetLabelI=on  LabelI=Ish1  Ipu=off  Pbase=100e6  Vbase=500e3  OutputType=Complex  PhasorSimulation=off  PSBequivalent=0
  Variable Load : Subsystem  mask(Variable Load (PQ Model)){Vn=MicroVol, Fn=fr, PF=1, Load0=20e3}
      mask prompts: Vn "Nominal L-L Voltage [Vrms]"; Fn "Nominal Frequency [Hz]"; PF "Power Factor [0 to 1]"; Load0 "Initial Load [W]"
      mask help:
      | The Variable Load block is a lumped approximation for a distribution feeder. For non-unity power factor loads, the input (active power) is scaled accordingly to generate a desired load.
      |
      | Note: The initial input load must be specified for use for Load Flow analysis.
      mask init:
      | P0 = Load0;
      | Q0 = Load0*sqrt(1/PF-1);
      mask Display:
      | image(imread('Residential.jpg'))
      | color('white')
      | port_label('input',1,'Load')
      | port_label('Rconn',1,'A')
      | port_label('Rconn',2,'B')
      | port_label('Rconn',3,'C')
  Variable Load1 : Subsystem  mask(Variable Load (PQ Model)){Vn=MicroVol, Fn=fr, PF=1, Load0=20e3}
      mask prompts: Vn "Nominal L-L Voltage [Vrms]"; Fn "Nominal Frequency [Hz]"; PF "Power Factor [0 to 1]"; Load0 "Initial Load [W]"
      mask help:
      | The Variable Load block is a lumped approximation for a distribution feeder. For non-unity power factor loads, the input (active power) is scaled accordingly to generate a desired load.
      |
      | Note: The initial input load must be specified for use for Load Flow analysis.
      mask init:
      | P0 = Load0;
      | Q0 = Load0*sqrt(1/PF-1);
      mask Display:
      | image(imread('Sharing.jpg'))
      | color('black')
      | % port_label('input',1,'Load')
      | port_label('Rconn',1,'A')
      | port_label('Rconn',2,'B')
      | port_label('Rconn',3,'C')
  A : PMIOPort  Side=Left
  B : PMIOPort  Port=2  Side=Left
  C : PMIOPort  Port=3  Side=Left
  tag scope: LoadMG1=global, SOCM1=global
  wires:
  Power Equation Wind Turbine (PQ Model)/1(m) -> [WTM]
  Solar Array/1(m) -> [Ppv]
  Constant2/1 -> Power Equation Wind Turbine (PQ Model)/2(Qref (pu))
  Load Profile MG1/1 -> Sum/1, Variable Load/1(Load)  "Load M1"
  Constant4/1 -> Simple Diesel Generator/2(Qref (pu))
  Simple Diesel Generator/1(m) -> Bus Selector1/1
  Bus Selector1/1 -> [PDG]  "<Active power P (W)>"
  Bus Selector1/2 -> Terminator/1  "<Reactive power Q (var)>"
  Gain5/1 -> Simple Diesel Generator/1(Pref (pu))
  Ref DG/1 -> Gain5/1
  Stair Generator1/1 -> Power Equation Wind Turbine (PQ Model)/1(Wind (m/s))
  Irradiation MG1/1 -> " "/1(Irra)
  Temeperature MG1/1 -> " "/2(Temp)
  " "/1(PowerOut) -> Solar Array/1(P)
  Active Power Dynamics1/1(Out) -> Energy Storage/1(Pref)
  Qref/1 -> Energy Storage/2(Qref)
  Energy Storage/2(Pbatt) -> [Pbb]
  Energy Storage/1(SOC (%)) -> [SOCM1]
  [LoadMG1] -> Scope/1(LOAD)  "Load M1"
  From37/1 -> Scope/2(VABC)
  From34/1 -> Scope/3(IABC)
  [PDG] -> Scope/4(PDG)
  [Pbb] -> Scope/5(PBB)
  [Ppv] -> Scope/6(PPV)
  [WTM] -> Scope/7(PWT)
  [VabcM1] -> "Power (3ph, Instantaneous)"/1
  [IabcM1] -> "Power (3ph, Instantaneous)"/2
  "Power (3ph, Instantaneous)"/1 -> Gain/1
  "Power (3ph, Instantaneous)"/2 -> Terminator1/1
  Gain/1 -> Scope1/1
  Sum/1 -> [LoadMG1]
  Constant/1 -> Sum/2
  Ref BB/1 -> Active Power Dynamics1/1(In)
  Gain1/1 -> Scope2/1
  "Power (3ph, Instantaneous)1"/2 -> Terminator2/1
  "Power (3ph, Instantaneous)1"/1 -> Gain1/1
  [Ish1] -> "Power (3ph, Instantaneous)1"/2
  [Vsh1] -> "Power (3ph, Instantaneous)1"/1
  connections:
  Simple Diesel Generator/LConn1 -- Load4/LConn1 -- Load3/LConn1 -- Power Equation Wind Turbine (PQ Model)/LConn1 -- Three-Phase V-I Measurement1/RConn1 -- Solar Array/RConn1 -- Load1/LConn1 -- Variable Load/RConn1 -- Load/LConn1 -- Three-Phase V-I Measurement2/RConn1 -- 1.5 Km Lines1/LConn1
  Three-Phase V-I Measurement2/LConn1 -- Load2/LConn1 -- Energy Storage/RConn1
  6 Km Lines/LConn1 -- Three-Phase Transformer (Two Windings)1/LConn1
  6 Km Lines/LConn3 -- Three-Phase Transformer (Two Windings)1/LConn3
  6 Km Lines/LConn2 -- Three-Phase Transformer (Two Windings)1/LConn2
  A/RConn1 -- 6 Km Lines/RConn1
  B/RConn1 -- 6 Km Lines/RConn2
  C/RConn1 -- 6 Km Lines/RConn3
  Three-Phase Transformer (Two Windings)1/RConn2 -- RL2/RConn2
  Three-Phase Transformer (Two Windings)1/RConn1 -- RL2/RConn1
  Three-Phase Transformer (Two Windings)1/RConn3 -- RL2/RConn3
  RL2/LConn1 -- Three-Phase V-I Measurement1/LConn1
  RL2/LConn2 -- Three-Phase V-I Measurement1/LConn2
  RL2/LConn3 -- Three-Phase V-I Measurement1/LConn3
  Three-Phase V-I Measurement2/LConn3 -- Load2/LConn3 -- Energy Storage/RConn3
  Energy Storage/RConn2 -- Load2/LConn2 -- Three-Phase V-I Measurement2/LConn2
  Simple Diesel Generator/LConn2 -- Load4/LConn2 -- Three-Phase V-I Measurement1/RConn2 -- Solar Array/RConn2 -- Load1/LConn2 -- Variable Load/RConn2 -- Load/LConn2 -- Three-Phase V-I Measurement2/RConn2 -- 1.5 Km Lines1/LConn2 -- Power Equation Wind Turbine (PQ Model)/LConn2 -- Load3/LConn2
  Variable Load1/RConn2 -- Three-Phase V-I Measurement3/RConn2
  Variable Load1/RConn1 -- Three-Phase V-I Measurement3/RConn1
  Variable Load1/RConn3 -- Three-Phase V-I Measurement3/RConn3
  Simple Diesel Generator/LConn3 -- Three-Phase V-I Measurement1/RConn3 -- Solar Array/RConn3 -- Load1/LConn3 -- Load/LConn3 -- Variable Load/RConn3 -- Three-Phase V-I Measurement2/RConn3 -- 1.5 Km Lines1/LConn3 -- Power Equation Wind Turbine (PQ Model)/LConn3 -- Load3/LConn3 -- Load4/LConn3
  Three-Phase V-I Measurement3/LConn1 -- 1.5 Km Lines1/RConn1
  Three-Phase V-I Measurement3/LConn2 -- 1.5 Km Lines1/RConn2
  Three-Phase V-I Measurement3/LConn3 -- 1.5 Km Lines1/RConn3
